simulink model "ModeloSimulacion2"  (R2023a)
settings: Solver=VariableStepAuto  StartTime=0.0  StopTime=40.0  RelTol=1e-3
values from neighbouring files (symbols this model uses):
  d = 0.02    [Simulacion2.m]
  G_g = pi/2    (= 1.57079632679)    [Simulacion2.m]
  G_x = 1    [Simulacion2.m]
  G_y = -1    [Simulacion2.m]
  J = 2    [Simulacion2.m]
  Kb = 1    [Simulacion2.m]
  Kt = 0.0300    (= 0.03)    [Simulacion2.m]
  L = 0.1    [Simulacion2.m]
  La = 0.94    [Simulacion2.m]
  M = 5    [Simulacion2.m]
  N = 1    [Simulacion2.m]
  R = 0.02    [Simulacion2.m]
  Ra = 1    [Simulacion2.m]
libraries: mobileRoboticsLib x1
settings Model: Creator=John_117  LastModifiedBy=John_117

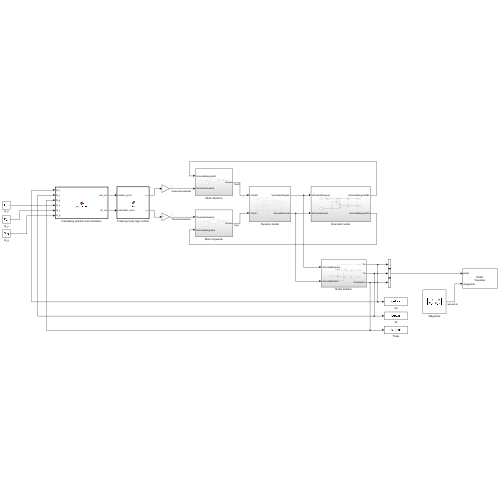
[thumbnail: Simulink's stored preview of the top-level diagram]
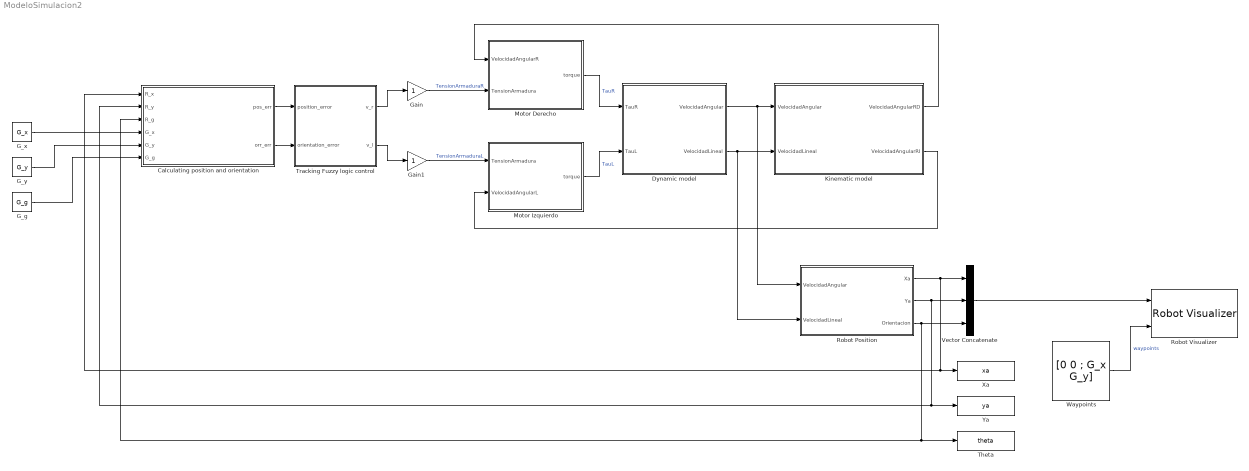
== system ModeloSimulacion2 ==
  Calculating position and orientation : MATLAB Function  TreatAsAtomicUnit=on
  Dynamic model : Subsystem
  G_g : Constant  Value=G_g
  G_x : Constant  Value=G_x
  G_y : Constant  Value=G_y
  Gain : Gain
  Gain1 : Gain
  Kinematic model : Subsystem
  Motor Derecho : Subsystem
  Motor Izquierdo : Subsystem
  Robot Position : Subsystem
  Robot Visualizer : mobileRoboticsLib/Environments/Robot Visualizer  robotRadius=0  showTrajectory=on  hasWaypoints=on  hasLidar=off  sensorOffset=[ 0, 0 ]  scanAngles=[ -pi/4, 0, pi/4 ]  hasObjDetector=off  objDetectorOffset=[ 0, 0 ]  objDetectorAngle=0  objDetectorFOV=pi/4  objDetectorMaxRange=5  objectColors=[ 1, 0, 0; 0, 1, 0; 0, 0, 1 ]  objectMarkers=s
  Theta : ToWorkspace  VariableName=theta  SaveFormat=Timeseries  SampleTime=-1
      settings: Save2DSignal=2-D array (concatenate along first dimension)
  Tracking Fuzzy logic control : MATLAB Function  TreatAsAtomicUnit=on
  Vector Concatenate : Concatenate  NumInputs=3
  Waypoints : Constant  Value="[0 0 ; G_x  G_y]"
  Xa : ToWorkspace  VariableName=xa  SaveFormat=Timeseries  SampleTime=-1
      settings: Save2DSignal=2-D array (concatenate along first dimension)
  Ya : ToWorkspace  VariableName=ya  SaveFormat=Timeseries  SampleTime=-1
      settings: Save2DSignal=2-D array (concatenate along first dimension)
  wires:
  Dynamic model/1(VelocidadAngular) -> Kinematic model/1(VelocidadAngular), Robot Position/1(VelocidadAngular)
  Dynamic model/2(VelocidadLineal) -> Kinematic model/2(VelocidadLineal), Robot Position/2(VelocidadLineal)
  Kinematic model/1(VelocidadAngularRD) -> Motor Derecho/1(VelocidadAngularR)
  Kinematic model/2(VelocidadAngularRI) -> Motor Izquierdo/2(VelocidadAngularL)
  Gain/1 -> Motor Derecho/2(TensionArmadura)  "TensionArmaduraR"
  Motor Derecho/1(torque) -> Dynamic model/1(TauR)  "TauR"
  Gain1/1 -> Motor Izquierdo/1(TensionArmadura)  "TensionArmaduraL"
  Motor Izquierdo/1(torque) -> Dynamic model/2(TauL)  "TauL"
  Robot Position/3(Orientacion) -> Theta/1, Calculating position and orientation/3(R_g), Vector Concatenate/3
  Robot Position/2(Ya) -> Ya/1, Calculating position and orientation/2(R_y), Vector Concatenate/2
  Vector Concatenate/1 -> Robot Visualizer/1
  Calculating position and orientation/2(orr_err) -> Tracking Fuzzy logic control/2(orientation_error)
  Calculating position and orientation/1(pos_err) -> Tracking Fuzzy logic control/1(position_error)
  Tracking Fuzzy logic control/1(v_r) -> Gain/1
  Tracking Fuzzy logic control/2(v_l) -> Gain1/1
  Robot Position/1(Xa) -> Vector Concatenate/1, Calculating position and orientation/1(R_x), Xa/1
  G_x/1 -> Calculating position and orientation/4(G_x)
  G_y/1 -> Calculating position and orientation/5(G_y)
  G_g/1 -> Calculating position and orientation/6(G_g)
  Waypoints/1 -> Robot Visualizer/2  "waypoints"

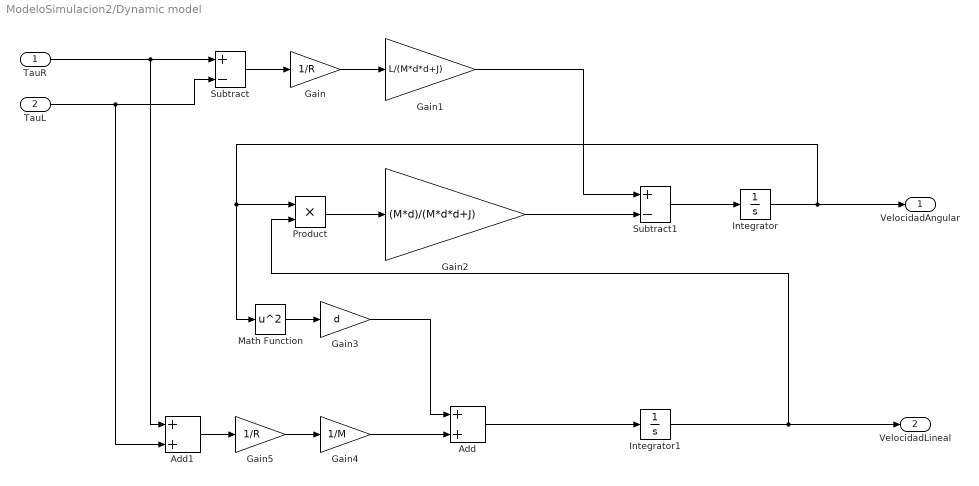
== system ModeloSimulacion2/Dynamic model ==
  TauR : Inport
  TauL : Inport  Port=2
  Add : Sum
  Add1 : Sum
  Gain : Gain  Gain=1/R
  Gain1 : Gain  Gain=L/(M*d*d+J)
  Gain2 : Gain  Gain=(M*d)/(M*d*d+J)
  Gain3 : Gain  Gain=d
  Gain4 : Gain  Gain=1/M
  Gain5 : Gain  Gain=1/R
  Integrator : Integrator
  Integrator1 : Integrator
  Math Function : Math  Operator=square
  Product : Product
  Subtract : Sum  Inputs=+-
  Subtract1 : Sum  Inputs=+-
  VelocidadAngular : Outport
  VelocidadLineal : Outport  Port=2
  wires:
  TauR/1 -> Add1/1, Subtract/1
  Gain4/1 -> Add/2
  Gain/1 -> Gain1/1
  Integrator/1 -> VelocidadAngular/1, Product/1, Math Function/1
  Integrator1/1 -> VelocidadLineal/1, Product/2
  Subtract1/1 -> Integrator/1
  Product/1 -> Gain2/1
  Gain1/1 -> Subtract1/1
  Gain5/1 -> Gain4/1
  Gain3/1 -> Add/1
  TauL/1 -> Add1/2, Subtract/2
  Math Function/1 -> Gain3/1
  Gain2/1 -> Subtract1/2
  Add1/1 -> Gain5/1
  Add/1 -> Integrator1/1
  Subtract/1 -> Gain/1

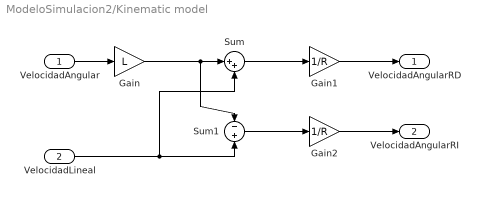
== system ModeloSimulacion2/Kinematic model ==
  VelocidadAngular : Inport
  VelocidadLineal : Inport  Port=2
  Gain : Gain  Gain=L
  Gain1 : Gain  Gain=1/R
  Gain2 : Gain  Gain=1/R
  Sum : Sum  Inputs=|++
  Sum1 : Sum  Inputs=-+
  VelocidadAngularRD : Outport
  VelocidadAngularRI : Outport  Port=2
  wires:
  Gain1/1 -> VelocidadAngularRD/1
  Sum1/1 -> Gain2/1
  Gain2/1 -> VelocidadAngularRI/1
  Gain/1 -> Sum/1, Sum1/1
  VelocidadLineal/1 -> Sum1/2, Sum/2
  VelocidadAngular/1 -> Gain/1
  Sum/1 -> Gain1/1

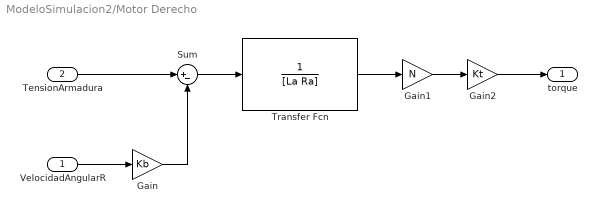
== system ModeloSimulacion2/Motor Derecho ==
  VelocidadAngularR : Inport
  TensionArmadura : Inport  Port=2
  Gain : Gain  Gain=Kb
  Gain1 : Gain  Gain=N
  Gain2 : Gain  Gain=Kt
  Sum : Sum  Inputs=|+-
  Transfer Fcn : TransferFcn  Denominator=[La Ra]
  torque : Outport
  wires:
  Sum/1 -> Transfer Fcn/1
  TensionArmadura/1 -> Sum/1
  Gain2/1 -> torque/1
  Gain/1 -> Sum/2
  Transfer Fcn/1 -> Gain1/1
  VelocidadAngularR/1 -> Gain/1
  Gain1/1 -> Gain2/1

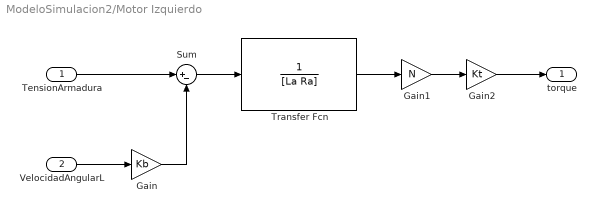
== system ModeloSimulacion2/Motor Izquierdo ==
  TensionArmadura : Inport
  VelocidadAngularL : Inport  Port=2
  Gain : Gain  Gain=Kb
  Gain1 : Gain  Gain=N
  Gain2 : Gain  Gain=Kt
  Sum : Sum  Inputs=|+-
  Transfer Fcn : TransferFcn  Denominator=[La Ra]
  torque : Outport
  wires:
  Sum/1 -> Transfer Fcn/1
  TensionArmadura/1 -> Sum/1
  Gain2/1 -> torque/1
  Gain/1 -> Sum/2
  Transfer Fcn/1 -> Gain1/1
  VelocidadAngularL/1 -> Gain/1
  Gain1/1 -> Gain2/1

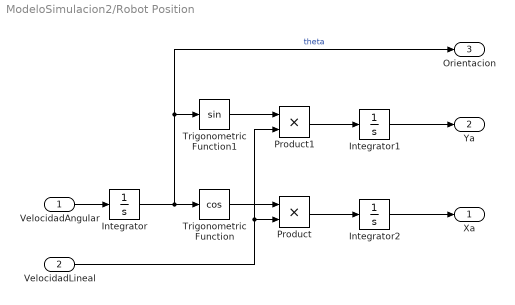
== system ModeloSimulacion2/Robot Position ==
  VelocidadAngular : Inport
  VelocidadLineal : Inport  Port=2
  Integrator : Integrator
  Integrator1 : Integrator
  Integrator2 : Integrator
  Product : Product
  Product1 : Product
  Trigonometric Function : Trigonometry  Operator=cos
  Trigonometric Function1 : Trigonometry
  Xa : Outport
  Ya : Outport  Port=2
  Orientacion : Outport  Port=3
  wires:
  Integrator1/1 -> Ya/1
  VelocidadAngular/1 -> Integrator/1
  Integrator2/1 -> Xa/1
  Integrator/1 -> Orientacion/1, Trigonometric Function1/1, Trigonometric Function/1  "theta"
  Product1/1 -> Integrator1/1
  Trigonometric Function/1 -> Product/1
  VelocidadLineal/1 -> Product1/2, Product/2
  Product/1 -> Integrator2/1
  Trigonometric Function1/1 -> Product1/1

== matlab function ModeloSimulacion2/Tracking Fuzzy logic control ==
  data: position_error input; v_r output; orientation_error input; v_l output
function [v_r,v_l] = tflc(position_error,orientation_error)
    %% global constant
    %TFLC RULES
    rules_TFLC_L = [
    1 1 1 1 3 3 4;
    2 2 1 2 3 5 6;
    2 2 2 3 5 6 7;
    1 1 1 4 6 6 7;
    2 2 3 5 5 6 7;
    1 1 4 6 5 6 7;
    2 2 3 7 5 6 7
    ];
    rules_TFLC_R = flip(rules_TFLC_L,2);
    %OAFLC RULES
    rules_OAFLC_R_L = [
    1 1; 2 1; 2 1; 1 1; 2 1; 2 1; 1 1; 2 1; 2 1;
    1 2; 1 1; 5 3; 3 5; 5 3; 5 3; 1 2; 5 3; 5 3;
    1 2; 3 5; 1 1; 1 2; 3 5; 5 3; 1 2; 3 5; 4 4;
    ];

    %% run all nested function
    %fuzzyfication
    fuz_dist = check_distance_membership(position_error); % in meter
    fuz_orie = check_err_angle_membership(orientation_error); % in degree angle
    %inference
    [mat_TFLC_L_rel,v_TFLC_L_th] = relate_TFLC (fuz_dist, fuz_orie, rules_TFLC_L);
    [mat_TFLC_R_rel,v_TFLC_R_th] = relate_TFLC (fuz_dist, fuz_orie, rules_TFLC_R);
    %calculating centroid TFLC L
    dt = 0.01;
    t = -1:dt:13; %output data range
    out = [];
    for i=1:length(t)
        ret=check_velocity_membership(t(i)); %output fuzzification
        ret = min(v_TFLC_L_th, ret);
        %Max value / real value of the inference
        out = [out max(ret)]; %MAX
    end
    centeroid_TFLC_L = sum(out.*t)/sum(out);
    %calculating centroid TFLC R
    out = [];
    for i=1:length(t)
        ret=check_velocity_membership(t(i)); %output fuzzification
        ret = min(v_TFLC_R_th, ret);
        %Max value / real value of the inference
        out = [out max(ret)]; %MAX
    end
    centeroid_TFLC_R = sum(out.*t)/sum(out);
    %actuate the wheel
    v_r = centeroid_TFLC_L; %because the rules is inverted
    v_l = centeroid_TFLC_R;
    
    %% %%%%%%%%%%%%%%%%%%%%%%%%%%%%%%%%%%%%%%%%%%%%%%%%%%%
    %%                      FUNCTIONS
    %% %%%%%%%%%%%%%%%%%%%%%%%%%%%%%%%%%%%%%%%%%%%%%%%%%%%
    %% =====================to check all value in distance fuzzification
    function out = check_distance_membership(input) %meter
        z = triangle (input, 0, 0, 0.50, 1, 1, 0); %zero
        nz = triangle (input, 0, 0.50, 1.00, 0, 1, 0); %near zero
        n = triangle (input, 0.50, 1.00, 1.50, 0, 1, 0); %near
        m = triangle (input, 1.00, 1.50, 2.00, 0, 1, 0); %medium
        nf = triangle (input, 1.50, 2.00, 2.50, 0, 1, 0); %near far
        f = triangle (input, 2.00, 2.50, 3.00, 0, 1, 0); %far
        vf = triangle (input, 2.50, 3.00, 3.00, 0, 1, 1); %very far
        out = [z;nz;n;m;nf;f;vf];
    end
    %% =====================to check all value in angle error fuzzification
    function out = check_err_angle_membership(input)
        n = triangle (input, -175, -175, -88, 1, 1, 0); %negative
        sn = triangle (input, -175, -88, -43, 0, 1, 0); %small neg
        nnz = triangle (input, -88, -43, 0, 0, 1, 0); % near neg zero
        z = triangle (input, -43, 0, 43, 0, 1, 0); %zero
        npz = triangle (input, 0, 43, 88, 0, 1, 0); %near pos zero
        sp = triangle (input, 43, 88, 175, 0, 1, 0); %small pos
        p = triangle (input, 88, 175, 175, 0, 1, 1); %positive
        out = [n; sn; nnz; z; npz; sp; p];
    end
    %% =====================to check all value in velocity of motors in TFLC fuzzification
    function out = check_velocity_membership(input)
        z = triangle (input, 0, 0, 2, 1, 1, 0);%zero
        s = triangle (input, 0, 2, 4, 0, 1, 0);%slow
        nm = triangle (input, 2, 4, 6, 0, 1, 0);%near medium
        m = triangle (input, 4, 6, 8, 0, 1, 0);%medium
        nh = triangle (input, 6, 8, 10, 0, 1, 0);%near high
        h = triangle (input, 8, 10, 12, 0, 1, 0);%high
        vh = triangle (input, 10, 12, 12, 0, 1, 1);%very high
        out = [z;s;nm;m;nh;h;vh];
    end
    %% ===============triangle shaped fuzzy membership
    function out = triangle (input, start, middle, stop, str_val, mid_val, sto_val)
        if input<start
            out = str_val;

        elseif (input>=start) && (input<middle)
            v = (mid_val-str_val)/(middle-start);
            out = str_val + v*(input-start);

        elseif (input==middle)
            out = mid_val;

        elseif (input>middle) && (input<=stop)
            v = (sto_val-mid_val)/(stop-middle);
            out = mid_val + v*(input-middle);

        elseif input>stop
            out = sto_val;
        else
            out = 0;
        end
    end
    %% Relate a fuzzification to another with the result of matrix & vec
    % the relation is using minimum, because the relation in fuzzy rules are
    % using AND
    function [mat_rules_val,v_out_th] = relate_TFLC (set1, set2, rules_index)
        % set1 is rows, and set2 is columns
        % find correspoding values for each rules
        m = zeros(length(set1), length(set2));
        for i=1:length(set1)
            for j=1:length(set2)
                m(i,j)=min(set1(i),set2(j)); %MIN
            end
        end

        % find the output index of each rules values
        % then create vector, of possible maximum mambership value from output
        % membership class
        v_out = zeros(max(max(rules_index)),1);
        [h,w]=size(rules_index);
        for i = 1:h
            for j = 1:w
                v_out( rules_index(i,j) ) = max(v_out( rules_index(i,j) ), m (i,j)); %MAX
            end
        end
        mat_rules_val = m;
        v_out_th = v_out;
    end
end

== matlab function ModeloSimulacion2/Calculating position and orientation ==
  data: R_x input; pos_err output; R_y input; R_g input; G_x input; G_y input; G_g input; orr_err output
function [pos_err,orr_err] = pos_orr_err(R_x, R_y, R_g, G_x, G_y, G_g)
    %values assignment
    rob_poss = [R_x; R_y]; %in meter
    gol_poss = [G_x; G_y]; %in meter
    gamma_r = R_g;         %in radian
%     % convert radian to -pi to pi values
%     if gamma_r>pi
%         gamma_r = gamma_r-2*pi;
%     elseif gamma_r<pi
%         gamma_r = gamma_r+2*pi;
%     end

    %position error
    vec_pos = gol_poss-rob_poss;
    pos_err = sqrt(sum((vec_pos).^2)); %in meter
    
    %Goal position relative to robot position to find heading error
    fTr = [cos(gamma_r) -sin(gamma_r) rob_poss(1); sin(gamma_r) cos(gamma_r) rob_poss(2); 0 0 1];
    gol_2_r_pos = (fTr)\[gol_poss(1); gol_poss(2); 1];
    %heading error
    hed_err = atan2(gol_2_r_pos(2), gol_2_r_pos(1));
    hed_err = rad2deg(hed_err);
    orr_err = hed_err; %in degree angle
end
